simulink model "trig"  (R2016a)
settings: Solver=VariableStepAuto  StartTime=0.0  StopTime=10.0  MaxStep=2^-7  RelTol=1e-3
libraries: simulink x1
settings Model: Creator=sk42595  LastModifiedBy=sk42595

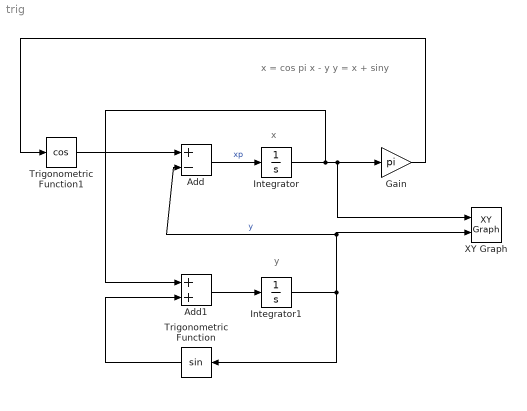
== system trig ==
  note: y
  note: x
  note: x = cos pi x - y
      | y = x + siny
  Add : Sum  Inputs=+-
  Add1 : Sum
  Gain : Gain  Gain=pi
  Integrator : Integrator  InitialCondition=70
  Integrator1 : Integrator  InitialCondition=1
  Trigonometric Function : Trigonometry
  Trigonometric Function1 : Trigonometry  Operator=cos
  XY Graph : simulink/Sinks/XY Graph  xmin=-80  xmax=80  ymin=-80  ymax=80  st=-1
  wires:
  Add1/1 -> Integrator1/1
  Add/1 -> Integrator/1  "xp"
  Integrator1/1 -> XY Graph/2, Add/2, Trigonometric Function/1  "y"
  Integrator/1 -> XY Graph/1, Gain/1, Add1/1
  Trigonometric Function/1 -> Add1/2
  Gain/1 -> Trigonometric Function1/1
  Trigonometric Function1/1 -> Add/1
